simulink model "ovap_sim"  (R2025a)
settings: Solver=FixedStepAuto  StartTime=0.0  StopTime=100  FixedStep=0.002  RelTol=1e-3
undefined symbols (not defined in the file): X, Y, Z
libraries: sm_lib x88, nesl_utility x45, simulink_extras x31, slpidlib x8
(part 3 of 5)

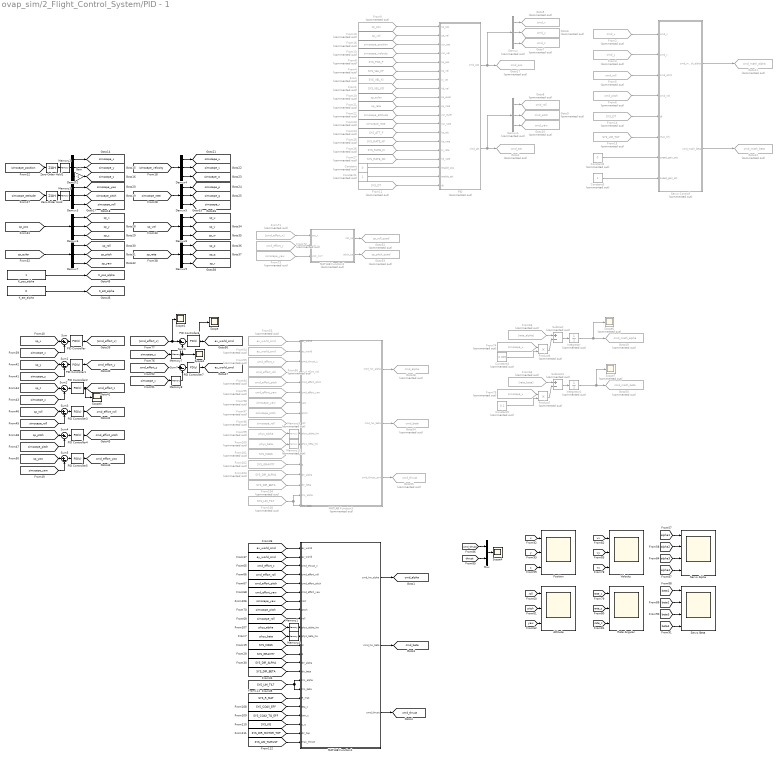
== system ovap_sim/2_Flight_Control_System/PID - 1 ==
  Attitude : Scope  NumInputPorts=3
      settings: ActiveDisplayYMinimum=-1.3426964874855616  ActiveDisplayYMaximum=11.260296121880314  DataLoggingVariableName=ScopeData17
  Constant : Constant  Commented=on  Value=0
  Constant1 : Constant  Commented=on
  Constant2 : Constant  Commented=on  Value=0
  Constant3 : Constant  Commented=on
  Constant4 : Constant  Commented=on  Value=0.005
  Constant5 : Constant  Commented=on  Value=0.1
  Demux : Demux  Commented=on  Outputs=3
  Demux1 : Demux  Commented=on  Outputs=3
  Demux{2..9} (8 alike) : Demux  Outputs=3
  From : From  Commented=on  GotoTag=SYS_VEL_KI  TagVisibility=global
  From1 : From  Commented=on  GotoTag=SYS_VEL_KD  TagVisibility=global
  From10 : From  Commented=on  GotoTag=sp_vel  TagVisibility=global
  From100 : From  Commented=on  GotoTag=phys_beta  TagVisibility=global
  From101 : From  Commented=on  GotoTag=SYS_MASS  TagVisibility=global
  From102 : From  Commented=on  GotoTag=SYS_GRAVITY  TagVisibility=global
  From103 : From  Commented=on  GotoTag=SYS_DIR_ALPHA  TagVisibility=global
  From104 : From  Commented=on  GotoTag=SYS_DIR_BETA  TagVisibility=global
  From105 : From  Commented=on  GotoTag=SYS_LIM_TILT  TagVisibility=global
  From11 : From  Commented=on  GotoTag=SYS_DT  TagVisibility=global
  From13 : From  Commented=on  GotoTag=simscape_velocity  TagVisibility=global
  From14 : From  Commented=on  GotoTag=SYS_DT  TagVisibility=global
  From15 : From  Commented=on  GotoTag=SYS_LIM_TILT  TagVisibility=global
  From16 : From  Commented=on  GotoTag=simscape_position  TagVisibility=global
  From2 : From  Commented=on  GotoTag=cmd_x  TagVisibility=global
  From20 : From  Commented=on  GotoTag=sp_euler  TagVisibility=global
  From21 : From  Commented=on  GotoTag=sp_rate  TagVisibility=global
  From22 : From  Commented=on  GotoTag=simscape_attitude  TagVisibility=global
  From23 : From  Commented=on  GotoTag=simscape_rate  TagVisibility=global
  From24 : From  Commented=on  GotoTag=SYS_ATT_P  TagVisibility=global
  From25 : From  Commented=on  GotoTag=SYS_RATE_KP  TagVisibility=global
  From26 : From  Commented=on  GotoTag=SYS_RATE_KI  TagVisibility=global
  From27 : From  Commented=on  GotoTag=SYS_RATE_KD  TagVisibility=global
  From3 : From  Commented=on  GotoTag=cmd_y  TagVisibility=global
  From4 : From  Commented=on  GotoTag=SYS_VEL_KP  TagVisibility=global
  From5 : From  Commented=on  GotoTag=cmd_roll  TagVisibility=global
  From53 : From  Commented=on  GotoTag=ax_world_cmd  TagVisibility=global
  From54 : From  Commented=on  GotoTag=ay_world_cmd  TagVisibility=global
  From55 : From  Commented=on  GotoTag=cmd_effort_z  TagVisibility=global
  From56 : From  Commented=on  GotoTag=cmd_effort_roll  TagVisibility=global
  From6 : From  Commented=on  GotoTag=cmd_pitch  TagVisibility=global
  From63 : From  Commented=on  GotoTag=rate_alpha
  From64 : From  Commented=on  GotoTag=rate_beta
  From71 : From  Commented=on  GotoTag=cmd_effort_x
  From72 : From  Commented=on  GotoTag=cmd_effort_y  TagVisibility=global
  From73 : From  Commented=on  GotoTag=simscape_yaw  TagVisibility=global
  From74 : From  Commented=on  GotoTag=simscape_u  TagVisibility=global
  From75 : From  Commented=on  GotoTag=simscape_v  TagVisibility=global
  From8 : From  Commented=on  GotoTag=SYS_POS_P  TagVisibility=global
  From9 : From  Commented=on  GotoTag=sp_pos  TagVisibility=global
  From94 : From  Commented=on  GotoTag=cmd_effort_pitch  TagVisibility=global
  From95 : From  Commented=on  GotoTag=cmd_effort_yaw  TagVisibility=global
  From96 : From  Commented=on  GotoTag=simscape_roll  TagVisibility=global
  From97 : From  Commented=on  GotoTag=simscape_pitch  TagVisibility=global
  From98 : From  Commented=on  GotoTag=simscape_yaw  TagVisibility=global
  From99 : From  Commented=on  GotoTag=phys_alpha  TagVisibility=global
  Gain : Gain  Gain=-1
  Goto10 : Goto  Commented=on  GotoTag=cmd_yaw  TagVisibility=global
  Goto11 : Goto  Commented=on  GotoTag=cmd_math_alpha  TagVisibility=global
  Goto12 : Goto  Commented=on  GotoTag=cmd_math_beta  TagVisibility=global
  Goto17 : Goto  Commented=on  GotoTag=cmd_pos  TagVisibility=global
  Goto2 : Goto  Commented=on  GotoTag=cmd_att  TagVisibility=global
  Goto48 : Goto  Commented=on  GotoTag=cmd_alpha  TagVisibility=global
  Goto49 : Goto  Commented=on  GotoTag=cmd_math_alpha  TagVisibility=global
  Goto5 : Goto  Commented=on  GotoTag=cmd_x  TagVisibility=global
  Goto50 : Goto  Commented=on  GotoTag=cmd_math_beta  TagVisibility=global
  Goto52 : Goto  Commented=on  GotoTag=sp_roll_quad  TagVisibility=global
  Goto53 : Goto  Commented=on  GotoTag=sp_pitch_quad  TagVisibility=global
  Goto54 : Goto  Commented=on  GotoTag=cmd_beta  TagVisibility=global
  Goto55 : Goto  Commented=on  GotoTag=cmd_thrust  TagVisibility=global
  Goto6 : Goto  Commented=on  GotoTag=cmd_y  TagVisibility=global
  Goto7 : Goto  Commented=on  GotoTag=cmd_z  TagVisibility=global
  Goto8 : Goto  Commented=on  GotoTag=cmd_roll  TagVisibility=global
  Goto9 : Goto  Commented=on  GotoTag=cmd_pitch  TagVisibility=global
  Integrator : Integrator  Commented=on  LimitOutput=on  UpperSaturationLimit=5*pi/180  LowerSaturationLimit=-5*pi/180
  Integrator1 : Integrator  Commented=on  LimitOutput=on  UpperSaturationLimit=5  LowerSaturationLimit=-5
  K_att_alpha : Constant  Value=0
  K_pos_alpha : Constant
  MATLAB Function1 : MATLAB Function  TreatAsAtomicUnit=on
  MATLAB Function2 : MATLAB Function  Commented=on  TreatAsAtomicUnit=on
  MATLAB Function3 : MATLAB Function  Commented=on  TreatAsAtomicUnit=on
  Memory{1..4,7..8} (6 alike) : Memory
  Memory10 : Memory  Commented=on
  Memory9 : Memory  Commented=on
  Mux : Mux  Inputs=2
  PID : MATLAB Function  Commented=on  TreatAsAtomicUnit=on
  PID Controller : slpidlib/PID Controller  Controller=PID  Form=Parallel  TimeDomain=Discrete-time  UseExternalTs=off  SampleTime=0.002  IntegratorMethod=Forward Euler  FilterMethod=Forward Euler  ControllerParametersSource=internal  P=15  I=0.0001  UseKiTs=off  D=27  UseExternalDerivativeSource=off  N=100  UseFilter=on  TunerSelectOption=Transfer Function Based (PID Tuner App)  InitialConditionSource=internal  InitialConditionForIntegrator=0  InitialConditionForFilter=0  DifferentiatorICPrevScaledInput=0  ExternalReset=none  TrackingMode=off  Kt=1  LimitOutput=off  SatLimitsSource=internal  UpperSaturationLimit=1  LowerSaturationLimit=-1  LinearizeAsGain=off  AntiWindupMode=clamping  Kb=1  LimitIntegrator=off  UpperIntegratorSaturationLimit=inf  LowerIntegratorSaturationLimit=-inf  POutMin=[]  POutMax=[]  IOutMin=[]  IOutMax=[]  DOutMin=[]  DOutMax=[]  NOutMin=[]  NOutMax=[]  SumOutMin=[]  SumOutMax=[]  SaturationOutMin=[]  SaturationOutMax=[]  PParamMin=[]  PParamMax=[]  IParamMin=[]  IParamMax=[]  DParamMin=[]  DParamMax=[]  NParamMin=[]  NParamMax=[]  KbParamMin=[]  KbParamMax=[]  KtParamMin=[]  KtParamMax=[]  KbOutMin=[]  KbOutMax=[]  KtOutMin=[]  KtOutMax=[]  IntegratorOutMin=[]  IntegratorOutMax=[]  FilterOutMin=[]  FilterOutMax=[]  SumI1OutMin=[]  SumI1OutMax=[]  SumI2OutMin=[]  SumI2OutMax=[]  SumI3OutMin=[]  SumI3OutMax=[]  SumI4OutMin=[]  SumI4OutMax=[]  SumDOutMin=[]  SumDOutMax=[]  DifferentiatorOutMin=[]  DifferentiatorOutMax=[]  FilterDiffOutCoefMin=[]  FilterDiffOutCoefMax=[]  ReciprocalOutMin=[]  ReciprocalOutMax=[]  SumDenOutMin=[]  SumDenOutMax=[]  SumNumOutMin=[]  SumNumOutMax=[]  DivideOutMin=[]  DivideOutMax=[]  UdiffTsProdOutMin=[]  UdiffTsProdOutMax=[]  NTsProdOutMin=[]  NTsProdOutMax=[]  UintegralTsProdOutMin=[]  UintegralTsProdOutMax=[]  UngainTsProdOutMin=[]  UngainTsProdOutMax=[]  ClampingZeroOutDataTypeStr=Inherit: Inherit via back propagation  ClampingZeroOutMin=[]  ClampingZeroOutMax=[]  FilterDenConstantOutDataTypeStr=Inherit: Inherit via back propagation  FilterDenConstantOutMin=[]  FilterDenConstantOutMax=[]  PCopyOutDataTypeStr=Inherit: Inherit via back propagation  PCopyOutMin=[]  PCopyOutMax=[]  NCopyOutDataTypeStr=Inherit: Inherit via back propagation  NCopyOutMin=[]  NCopyOutMax=[]  IntegratorContinuousStateAttributes=''  IntegratorStateMustResolveToSignalObject=off  IntegratorRTWStateStorageClass=Auto  FilterContinuousStateAttributes=''  FilterStateMustResolveToSignalObject=off  FilterRTWStateStorageClass=Auto  ParallelPVariant=InternalParameters  IdealPVariant=Disabled  IVariant=InternalParameters  DVariant=InternalParameters  IntegratorVariant=Discrete  SatVariant=Disabled  AWVariant=Passthrough  PCopyVariant=Disabled  TRVariant=Disabled  FdbkBlocksVariant=Forward  IdealPFdbkVariant=Disabled  SatFdbkVariant=Disabled  DerivativeFilterVariant=ForwardEulerFilter  NVariant=InternalParameters  NCopyVariant=Disabled  FilterICVariant=InternalICsFilter  IntegratorICVariant=InternalICs  ExternalResetVariant=Disabled  TRSumVariant=Passthrough  SumFdbkVariant=Disabled  SumVariant=Sum_PID  TsampFilterVariant=InternalTs  TsampNgainVariant=Passthrough  TsampIntegralVariant=Disabled_SignalSpec  ExternalSaturationOutDataTypeStr=Inherit: Same as second input  DerivativeSourceVariant=ErrorSignal  PreIntVariant=InternalPreInt
  PID Controller1 : slpidlib/PID Controller  Controller=PID  Form=Parallel  TimeDomain=Discrete-time  UseExternalTs=off  SampleTime=0.002  IntegratorMethod=Forward Euler  FilterMethod=Forward Euler  ControllerParametersSource=internal  P=3  I=0.0001  UseKiTs=off  D=0  UseExternalDerivativeSource=off  N=100  UseFilter=on  TunerSelectOption=Transfer Function Based (PID Tuner App)  InitialConditionSource=internal  InitialConditionForIntegrator=0  InitialConditionForFilter=0  DifferentiatorICPrevScaledInput=0  ExternalReset=none  TrackingMode=off  Kt=1  LimitOutput=on  SatLimitsSource=internal  UpperSaturationLimit=5  LowerSaturationLimit=-5  LinearizeAsGain=on  AntiWindupMode=clamping  Kb=1  LimitIntegrator=off  UpperIntegratorSaturationLimit=inf  LowerIntegratorSaturationLimit=-inf  POutMin=[]  POutMax=[]  IOutMin=[]  IOutMax=[]  DOutMin=[]  DOutMax=[]  NOutMin=[]  NOutMax=[]  SumOutMin=[]  SumOutMax=[]  SaturationOutMin=[]  SaturationOutMax=[]  PParamMin=[]  PParamMax=[]  IParamMin=[]  IParamMax=[]  DParamMin=[]  DParamMax=[]  NParamMin=[]  NParamMax=[]  KbParamMin=[]  KbParamMax=[]  KtParamMin=[]  KtParamMax=[]  KbOutMin=[]  KbOutMax=[]  KtOutMin=[]  KtOutMax=[]  IntegratorOutMin=[]  IntegratorOutMax=[]  FilterOutMin=[]  FilterOutMax=[]  SumI1OutMin=[]  SumI1OutMax=[]  SumI2OutMin=[]  SumI2OutMax=[]  SumI3OutMin=[]  SumI3OutMax=[]  SumI4OutMin=[]  SumI4OutMax=[]  SumDOutMin=[]  SumDOutMax=[]  DifferentiatorOutMin=[]  DifferentiatorOutMax=[]  FilterDiffOutCoefMin=[]  FilterDiffOutCoefMax=[]  ReciprocalOutMin=[]  ReciprocalOutMax=[]  SumDenOutMin=[]  SumDenOutMax=[]  SumNumOutMin=[]  SumNumOutMax=[]  DivideOutMin=[]  DivideOutMax=[]  UdiffTsProdOutMin=[]  UdiffTsProdOutMax=[]  NTsProdOutMin=[]  NTsProdOutMax=[]  UintegralTsProdOutMin=[]  UintegralTsProdOutMax=[]  UngainTsProdOutMin=[]  UngainTsProdOutMax=[]  ClampingZeroOutDataTypeStr=Inherit: Inherit via back propagation  ClampingZeroOutMin=[]  ClampingZeroOutMax=[]  FilterDenConstantOutDataTypeStr=Inherit: Inherit via back propagation  FilterDenConstantOutMin=[]  FilterDenConstantOutMax=[]  PCopyOutDataTypeStr=Inherit: Inherit via back propagation  PCopyOutMin=[]  PCopyOutMax=[]  NCopyOutDataTypeStr=Inherit: Inherit via back propagation  NCopyOutMin=[]  NCopyOutMax=[]  IntegratorContinuousStateAttributes=''  IntegratorStateMustResolveToSignalObject=off  IntegratorRTWStateStorageClass=Auto  FilterContinuousStateAttributes=''  FilterStateMustResolveToSignalObject=off  FilterRTWStateStorageClass=Auto  ParallelPVariant=InternalParameters  IdealPVariant=Disabled  IVariant=InternalParameters  DVariant=InternalParameters  IntegratorVariant=Discrete  SatVariant=Enabled  AWVariant=DiscClampingParallel  PCopyVariant=Disabled  TRVariant=Disabled  FdbkBlocksVariant=Forward  IdealPFdbkVariant=Disabled  SatFdbkVariant=Disabled  DerivativeFilterVariant=ForwardEulerFilter  NVariant=InternalParameters  NCopyVariant=Disabled  FilterICVariant=InternalICsFilter  IntegratorICVariant=InternalICs  ExternalResetVariant=Disabled  TRSumVariant=Passthrough  SumFdbkVariant=Disabled  SumVariant=Sum_PID  TsampFilterVariant=InternalTs  TsampNgainVariant=Passthrough  TsampIntegralVariant=Disabled_SignalSpec  ExternalSaturationOutDataTypeStr=Inherit: Same as second input  DerivativeSourceVariant=ErrorSignal  PreIntVariant=InternalPreInt
  PID Controller2 : slpidlib/PID Controller  Controller=PID  Form=Parallel  TimeDomain=Discrete-time  UseExternalTs=off  SampleTime=0.002  IntegratorMethod=Forward Euler  FilterMethod=Forward Euler  ControllerParametersSource=internal  P=3  I=0.0001  UseKiTs=off  D=9.5  UseExternalDerivativeSource=off  N=100  UseFilter=on  TunerSelectOption=Transfer Function Based (PID Tuner App)  InitialConditionSource=internal  InitialConditionForIntegrator=0  InitialConditionForFilter=0  DifferentiatorICPrevScaledInput=0  ExternalReset=none  TrackingMode=off  Kt=1  LimitOutput=on  SatLimitsSource=internal  UpperSaturationLimit=5  LowerSaturationLimit=-5  LinearizeAsGain=on  AntiWindupMode=clamping  Kb=1  LimitIntegrator=off  UpperIntegratorSaturationLimit=inf  LowerIntegratorSaturationLimit=-inf  POutMin=[]  POutMax=[]  IOutMin=[]  IOutMax=[]  DOutMin=[]  DOutMax=[]  NOutMin=[]  NOutMax=[]  SumOutMin=[]  SumOutMax=[]  SaturationOutMin=[]  SaturationOutMax=[]  PParamMin=[]  PParamMax=[]  IParamMin=[]  IParamMax=[]  DParamMin=[]  DParamMax=[]  NParamMin=[]  NParamMax=[]  KbParamMin=[]  KbParamMax=[]  KtParamMin=[]  KtParamMax=[]  KbOutMin=[]  KbOutMax=[]  KtOutMin=[]  KtOutMax=[]  IntegratorOutMin=[]  IntegratorOutMax=[]  FilterOutMin=[]  FilterOutMax=[]  SumI1OutMin=[]  SumI1OutMax=[]  SumI2OutMin=[]  SumI2OutMax=[]  SumI3OutMin=[]  SumI3OutMax=[]  SumI4OutMin=[]  SumI4OutMax=[]  SumDOutMin=[]  SumDOutMax=[]  DifferentiatorOutMin=[]  DifferentiatorOutMax=[]  FilterDiffOutCoefMin=[]  FilterDiffOutCoefMax=[]  ReciprocalOutMin=[]  ReciprocalOutMax=[]  SumDenOutMin=[]  SumDenOutMax=[]  SumNumOutMin=[]  SumNumOutMax=[]  DivideOutMin=[]  DivideOutMax=[]  UdiffTsProdOutMin=[]  UdiffTsProdOutMax=[]  NTsProdOutMin=[]  NTsProdOutMax=[]  UintegralTsProdOutMin=[]  UintegralTsProdOutMax=[]  UngainTsProdOutMin=[]  UngainTsProdOutMax=[]  ClampingZeroOutDataTypeStr=Inherit: Inherit via back propagation  ClampingZeroOutMin=[]  ClampingZeroOutMax=[]  FilterDenConstantOutDataTypeStr=Inherit: Inherit via back propagation  FilterDenConstantOutMin=[]  FilterDenConstantOutMax=[]  PCopyOutDataTypeStr=Inherit: Inherit via back propagation  PCopyOutMin=[]  PCopyOutMax=[]  NCopyOutDataTypeStr=Inherit: Inherit via back propagation  NCopyOutMin=[]  NCopyOutMax=[]  IntegratorContinuousStateAttributes=''  IntegratorStateMustResolveToSignalObject=off  IntegratorRTWStateStorageClass=Auto  FilterContinuousStateAttributes=''  FilterStateMustResolveToSignalObject=off  FilterRTWStateStorageClass=Auto  ParallelPVariant=InternalParameters  IdealPVariant=Disabled  IVariant=InternalParameters  DVariant=InternalParameters  IntegratorVariant=Discrete  SatVariant=Enabled  AWVariant=DiscClampingParallel  PCopyVariant=Disabled  TRVariant=Disabled  FdbkBlocksVariant=Forward  IdealPFdbkVariant=Disabled  SatFdbkVariant=Disabled  DerivativeFilterVariant=ForwardEulerFilter  NVariant=InternalParameters  NCopyVariant=Disabled  FilterICVariant=InternalICsFilter  IntegratorICVariant=InternalICs  ExternalResetVariant=Disabled  TRSumVariant=Passthrough  SumFdbkVariant=Disabled  SumVariant=Sum_PID  TsampFilterVariant=InternalTs  TsampNgainVariant=Passthrough  TsampIntegralVariant=Disabled_SignalSpec  ExternalSaturationOutDataTypeStr=Inherit: Same as second input  DerivativeSourceVariant=ErrorSignal  PreIntVariant=InternalPreInt
  PID Controller3 : slpidlib/PID Controller  Controller=PID  Form=Parallel  TimeDomain=Discrete-time  UseExternalTs=off  SampleTime=0.002  IntegratorMethod=Forward Euler  FilterMethod=Forward Euler  ControllerParametersSource=internal  P=0.05  I=0.0001  UseKiTs=off  D=0.4  UseExternalDerivativeSource=off  N=100  UseFilter=on  TunerSelectOption=Transfer Function Based (PID Tuner App)  InitialConditionSource=internal  InitialConditionForIntegrator=0  InitialConditionForFilter=0  DifferentiatorICPrevScaledInput=0  ExternalReset=none  TrackingMode=off  Kt=1  LimitOutput=on  SatLimitsSource=internal  UpperSaturationLimit=5  LowerSaturationLimit=-5  LinearizeAsGain=on  AntiWindupMode=none  Kb=1  LimitIntegrator=off  UpperIntegratorSaturationLimit=inf  LowerIntegratorSaturationLimit=-inf  POutMin=[]  POutMax=[]  IOutMin=[]  IOutMax=[]  DOutMin=[]  DOutMax=[]  NOutMin=[]  NOutMax=[]  SumOutMin=[]  SumOutMax=[]  SaturationOutMin=[]  SaturationOutMax=[]  PParamMin=[]  PParamMax=[]  IParamMin=[]  IParamMax=[]  DParamMin=[]  DParamMax=[]  NParamMin=[]  NParamMax=[]  KbParamMin=[]  KbParamMax=[]  KtParamMin=[]  KtParamMax=[]  KbOutMin=[]  KbOutMax=[]  KtOutMin=[]  KtOutMax=[]  IntegratorOutMin=[]  IntegratorOutMax=[]  FilterOutMin=[]  FilterOutMax=[]  SumI1OutMin=[]  SumI1OutMax=[]  SumI2OutMin=[]  SumI2OutMax=[]  SumI3OutMin=[]  SumI3OutMax=[]  SumI4OutMin=[]  SumI4OutMax=[]  SumDOutMin=[]  SumDOutMax=[]  DifferentiatorOutMin=[]  DifferentiatorOutMax=[]  FilterDiffOutCoefMin=[]  FilterDiffOutCoefMax=[]  ReciprocalOutMin=[]  ReciprocalOutMax=[]  SumDenOutMin=[]  SumDenOutMax=[]  SumNumOutMin=[]  SumNumOutMax=[]  DivideOutMin=[]  DivideOutMax=[]  UdiffTsProdOutMin=[]  UdiffTsProdOutMax=[]  NTsProdOutMin=[]  NTsProdOutMax=[]  UintegralTsProdOutMin=[]  UintegralTsProdOutMax=[]  UngainTsProdOutMin=[]  UngainTsProdOutMax=[]  ClampingZeroOutDataTypeStr=Inherit: Inherit via back propagation  ClampingZeroOutMin=[]  ClampingZeroOutMax=[]  FilterDenConstantOutDataTypeStr=Inherit: Inherit via back propagation  FilterDenConstantOutMin=[]  FilterDenConstantOutMax=[]  PCopyOutDataTypeStr=Inherit: Inherit via back propagation  PCopyOutMin=[]  PCopyOutMax=[]  NCopyOutDataTypeStr=Inherit: Inherit via back propagation  NCopyOutMin=[]  NCopyOutMax=[]  IntegratorContinuousStateAttributes=''  IntegratorStateMustResolveToSignalObject=off  IntegratorRTWStateStorageClass=Auto  FilterContinuousStateAttributes=''  FilterStateMustResolveToSignalObject=off  FilterRTWStateStorageClass=Auto  ParallelPVariant=InternalParameters  IdealPVariant=Disabled  IVariant=InternalParameters  DVariant=InternalParameters  IntegratorVariant=Discrete  SatVariant=Enabled  AWVariant=Passthrough  PCopyVariant=Disabled  TRVariant=Disabled  FdbkBlocksVariant=Forward  IdealPFdbkVariant=Disabled  SatFdbkVariant=Disabled  DerivativeFilterVariant=ForwardEulerFilter  NVariant=InternalParameters  NCopyVariant=Disabled  FilterICVariant=InternalICsFilter  IntegratorICVariant=InternalICs  ExternalResetVariant=Disabled  TRSumVariant=Passthrough  SumFdbkVariant=Disabled  SumVariant=Sum_PID  TsampFilterVariant=InternalTs  TsampNgainVariant=Passthrough  TsampIntegralVariant=Disabled_SignalSpec  ExternalSaturationOutDataTypeStr=Inherit: Same as second input  DerivativeSourceVariant=ErrorSignal  PreIntVariant=InternalPreInt
  PID Controller4 : slpidlib/PID Controller  Controller=PID  Form=Parallel  TimeDomain=Discrete-time  UseExternalTs=off  SampleTime=0.002  IntegratorMethod=Forward Euler  FilterMethod=Forward Euler  ControllerParametersSource=internal  P=0.06  I=0.00012  UseKiTs=off  D=0.68  UseExternalDerivativeSource=off  N=100  UseFilter=on  TunerSelectOption=Transfer Function Based (PID Tuner App)  InitialConditionSource=internal  InitialConditionForIntegrator=0  InitialConditionForFilter=0  DifferentiatorICPrevScaledInput=0  ExternalReset=none  TrackingMode=off  Kt=1  LimitOutput=on  SatLimitsSource=internal  UpperSaturationLimit=5  LowerSaturationLimit=-5  LinearizeAsGain=on  AntiWindupMode=none  Kb=1  LimitIntegrator=off  UpperIntegratorSaturationLimit=inf  LowerIntegratorSaturationLimit=-inf  POutMin=[]  POutMax=[]  IOutMin=[]  IOutMax=[]  DOutMin=[]  DOutMax=[]  NOutMin=[]  NOutMax=[]  SumOutMin=[]  SumOutMax=[]  SaturationOutMin=[]  SaturationOutMax=[]  PParamMin=[]  PParamMax=[]  IParamMin=[]  IParamMax=[]  DParamMin=[]  DParamMax=[]  NParamMin=[]  NParamMax=[]  KbParamMin=[]  KbParamMax=[]  KtParamMin=[]  KtParamMax=[]  KbOutMin=[]  KbOutMax=[]  KtOutMin=[]  KtOutMax=[]  IntegratorOutMin=[]  IntegratorOutMax=[]  FilterOutMin=[]  FilterOutMax=[]  SumI1OutMin=[]  SumI1OutMax=[]  SumI2OutMin=[]  SumI2OutMax=[]  SumI3OutMin=[]  SumI3OutMax=[]  SumI4OutMin=[]  SumI4OutMax=[]  SumDOutMin=[]  SumDOutMax=[]  DifferentiatorOutMin=[]  DifferentiatorOutMax=[]  FilterDiffOutCoefMin=[]  FilterDiffOutCoefMax=[]  ReciprocalOutMin=[]  ReciprocalOutMax=[]  SumDenOutMin=[]  SumDenOutMax=[]  SumNumOutMin=[]  SumNumOutMax=[]  DivideOutMin=[]  DivideOutMax=[]  UdiffTsProdOutMin=[]  UdiffTsProdOutMax=[]  NTsProdOutMin=[]  NTsProdOutMax=[]  UintegralTsProdOutMin=[]  UintegralTsProdOutMax=[]  UngainTsProdOutMin=[]  UngainTsProdOutMax=[]  ClampingZeroOutDataTypeStr=Inherit: Inherit via back propagation  ClampingZeroOutMin=[]  ClampingZeroOutMax=[]  FilterDenConstantOutDataTypeStr=Inherit: Inherit via back propagation  FilterDenConstantOutMin=[]  FilterDenConstantOutMax=[]  PCopyOutDataTypeStr=Inherit: Inherit via back propagation  PCopyOutMin=[]  PCopyOutMax=[]  NCopyOutDataTypeStr=Inherit: Inherit via back propagation  NCopyOutMin=[]  NCopyOutMax=[]  IntegratorContinuousStateAttributes=''  IntegratorStateMustResolveToSignalObject=off  IntegratorRTWStateStorageClass=Auto  FilterContinuousStateAttributes=''  FilterStateMustResolveToSignalObject=off  FilterRTWStateStorageClass=Auto  ParallelPVariant=InternalParameters  IdealPVariant=Disabled  IVariant=InternalParameters  DVariant=InternalParameters  IntegratorVariant=Discrete  SatVariant=Enabled  AWVariant=Passthrough  PCopyVariant=Disabled  TRVariant=Disabled  FdbkBlocksVariant=Forward  IdealPFdbkVariant=Disabled  SatFdbkVariant=Disabled  DerivativeFilterVariant=ForwardEulerFilter  NVariant=InternalParameters  NCopyVariant=Disabled  FilterICVariant=InternalICsFilter  IntegratorICVariant=InternalICs  ExternalResetVariant=Disabled  TRSumVariant=Passthrough  SumFdbkVariant=Disabled  SumVariant=Sum_PID  TsampFilterVariant=InternalTs  TsampNgainVariant=Passthrough  TsampIntegralVariant=Disabled_SignalSpec  ExternalSaturationOutDataTypeStr=Inherit: Same as second input  DerivativeSourceVariant=ErrorSignal  PreIntVariant=InternalPreInt
  PID Controller5 : slpidlib/PID Controller  Controller=PID  Form=Parallel  TimeDomain=Discrete-time  UseExternalTs=off  SampleTime=0.002  IntegratorMethod=Forward Euler  FilterMethod=Forward Euler  ControllerParametersSource=internal  P=2  I=0.0001  UseKiTs=off  D=16  UseExternalDerivativeSource=off  N=100  UseFilter=on  TunerSelectOption=Transfer Function Based (PID Tuner App)  InitialConditionSource=internal  InitialConditionForIntegrator=0  InitialConditionForFilter=0  DifferentiatorICPrevScaledInput=0  ExternalReset=none  TrackingMode=off  Kt=1  LimitOutput=on  SatLimitsSource=internal  UpperSaturationLimit=5  LowerSaturationLimit=-5  LinearizeAsGain=on  AntiWindupMode=none  Kb=1  LimitIntegrator=off  UpperIntegratorSaturationLimit=inf  LowerIntegratorSaturationLimit=-inf  POutMin=[]  POutMax=[]  IOutMin=[]  IOutMax=[]  DOutMin=[]  DOutMax=[]  NOutMin=[]  NOutMax=[]  SumOutMin=[]  SumOutMax=[]  SaturationOutMin=[]  SaturationOutMax=[]  PParamMin=[]  PParamMax=[]  IParamMin=[]  IParamMax=[]  DParamMin=[]  DParamMax=[]  NParamMin=[]  NParamMax=[]  KbParamMin=[]  KbParamMax=[]  KtParamMin=[]  KtParamMax=[]  KbOutMin=[]  KbOutMax=[]  KtOutMin=[]  KtOutMax=[]  IntegratorOutMin=[]  IntegratorOutMax=[]  FilterOutMin=[]  FilterOutMax=[]  SumI1OutMin=[]  SumI1OutMax=[]  SumI2OutMin=[]  SumI2OutMax=[]  SumI3OutMin=[]  SumI3OutMax=[]  SumI4OutMin=[]  SumI4OutMax=[]  SumDOutMin=[]  SumDOutMax=[]  DifferentiatorOutMin=[]  DifferentiatorOutMax=[]  FilterDiffOutCoefMin=[]  FilterDiffOutCoefMax=[]  ReciprocalOutMin=[]  ReciprocalOutMax=[]  SumDenOutMin=[]  SumDenOutMax=[]  SumNumOutMin=[]  SumNumOutMax=[]  DivideOutMin=[]  DivideOutMax=[]  UdiffTsProdOutMin=[]  UdiffTsProdOutMax=[]  NTsProdOutMin=[]  NTsProdOutMax=[]  UintegralTsProdOutMin=[]  UintegralTsProdOutMax=[]  UngainTsProdOutMin=[]  UngainTsProdOutMax=[]  ClampingZeroOutDataTypeStr=Inherit: Inherit via back propagation  ClampingZeroOutMin=[]  ClampingZeroOutMax=[]  FilterDenConstantOutDataTypeStr=Inherit: Inherit via back propagation  FilterDenConstantOutMin=[]  FilterDenConstantOutMax=[]  PCopyOutDataTypeStr=Inherit: Inherit via back propagation  PCopyOutMin=[]  PCopyOutMax=[]  NCopyOutDataTypeStr=Inherit: Inherit via back propagation  NCopyOutMin=[]  NCopyOutMax=[]  IntegratorContinuousStateAttributes=''  IntegratorStateMustResolveToSignalObject=off  IntegratorRTWStateStorageClass=Auto  FilterContinuousStateAttributes=''  FilterStateMustResolveToSignalObject=off  FilterRTWStateStorageClass=Auto  ParallelPVariant=InternalParameters  IdealPVariant=Disabled  IVariant=InternalParameters  DVariant=InternalParameters  IntegratorVariant=Discrete  SatVariant=Enabled  AWVariant=Passthrough  PCopyVariant=Disabled  TRVariant=Disabled  FdbkBlocksVariant=Forward  IdealPFdbkVariant=Disabled  SatFdbkVariant=Disabled  DerivativeFilterVariant=ForwardEulerFilter  NVariant=InternalParameters  NCopyVariant=Disabled  FilterICVariant=InternalICsFilter  IntegratorICVariant=InternalICs  ExternalResetVariant=Disabled  TRSumVariant=Passthrough  SumFdbkVariant=Disabled  SumVariant=Sum_PID  TsampFilterVariant=InternalTs  TsampNgainVariant=Passthrough  TsampIntegralVariant=Disabled_SignalSpec  ExternalSaturationOutDataTypeStr=Inherit: Same as second input  DerivativeSourceVariant=ErrorSignal  PreIntVariant=InternalPreInt
  PID Controller6 : slpidlib/PID Controller  Controller=PD  Form=Parallel  TimeDomain=Discrete-time  UseExternalTs=off  SampleTime=0.002  IntegratorMethod=Forward Euler  FilterMethod=Forward Euler  ControllerParametersSource=internal  P=1  I=0  UseKiTs=off  D=0.05  UseExternalDerivativeSource=off  N=100  UseFilter=on  TunerSelectOption=Transfer Function Based (PID Tuner App)  InitialConditionSource=internal  InitialConditionForIntegrator=0  InitialConditionForFilter=0  DifferentiatorICPrevScaledInput=0  ExternalReset=none  TrackingMode=off  Kt=1  LimitOutput=on  SatLimitsSource=internal  UpperSaturationLimit=3  LowerSaturationLimit=-3  LinearizeAsGain=off  AntiWindupMode=clamping  Kb=1  LimitIntegrator=off  UpperIntegratorSaturationLimit=inf  LowerIntegratorSaturationLimit=-inf  POutMin=[]  POutMax=[]  IOutMin=[]  IOutMax=[]  DOutMin=[]  DOutMax=[]  NOutMin=[]  NOutMax=[]  SumOutMin=[]  SumOutMax=[]  SaturationOutMin=[]  SaturationOutMax=[]  PParamMin=[]  PParamMax=[]  IParamMin=[]  IParamMax=[]  DParamMin=[]  DParamMax=[]  NParamMin=[]  NParamMax=[]  KbParamMin=[]  KbParamMax=[]  KtParamMin=[]  KtParamMax=[]  KbOutMin=[]  KbOutMax=[]  KtOutMin=[]  KtOutMax=[]  IntegratorOutMin=[]  IntegratorOutMax=[]  FilterOutMin=[]  FilterOutMax=[]  SumI1OutMin=[]  SumI1OutMax=[]  SumI2OutMin=[]  SumI2OutMax=[]  SumI3OutMin=[]  SumI3OutMax=[]  SumI4OutMin=[]  SumI4OutMax=[]  SumDOutMin=[]  SumDOutMax=[]  DifferentiatorOutMin=[]  DifferentiatorOutMax=[]  FilterDiffOutCoefMin=[]  FilterDiffOutCoefMax=[]  ReciprocalOutMin=[]  ReciprocalOutMax=[]  SumDenOutMin=[]  SumDenOutMax=[]  SumNumOutMin=[]  SumNumOutMax=[]  DivideOutMin=[]  DivideOutMax=[]  UdiffTsProdOutMin=[]  UdiffTsProdOutMax=[]  NTsProdOutMin=[]  NTsProdOutMax=[]  UintegralTsProdOutMin=[]  UintegralTsProdOutMax=[]  UngainTsProdOutMin=[]  UngainTsProdOutMax=[]  ClampingZeroOutDataTypeStr=Inherit: Inherit via back propagation  ClampingZeroOutMin=[]  ClampingZeroOutMax=[]  FilterDenConstantOutDataTypeStr=Inherit: Inherit via back propagation  FilterDenConstantOutMin=[]  FilterDenConstantOutMax=[]  PCopyOutDataTypeStr=Inherit: Inherit via back propagation  PCopyOutMin=[]  PCopyOutMax=[]  NCopyOutDataTypeStr=Inherit: Inherit via back propagation  NCopyOutMin=[]  NCopyOutMax=[]  IntegratorContinuousStateAttributes=''  IntegratorStateMustResolveToSignalObject=off  IntegratorRTWStateStorageClass=Auto  FilterContinuousStateAttributes=''  FilterStateMustResolveToSignalObject=off  FilterRTWStateStorageClass=Auto  ParallelPVariant=InternalParameters  IdealPVariant=Disabled  IVariant=Disabled  DVariant=InternalParameters  IntegratorVariant=Disabled  SatVariant=Enabled  AWVariant=Disabled  PCopyVariant=Disabled  TRVariant=Disabled  FdbkBlocksVariant=Forward  IdealPFdbkVariant=Disabled  SatFdbkVariant=Disabled  DerivativeFilterVariant=ForwardEulerFilter  NVariant=InternalParameters  NCopyVariant=Disabled  FilterICVariant=InternalICsFilter  IntegratorICVariant=Disabled  ExternalResetVariant=Disabled  TRSumVariant=Passthrough  SumFdbkVariant=Disabled  SumVariant=Sum_PD  TsampFilterVariant=InternalTs  TsampNgainVariant=Passthrough  TsampIntegralVariant=Disabled_SignalSpec  ExternalSaturationOutDataTypeStr=Inherit: Same as second input  DerivativeSourceVariant=ErrorSignal  PreIntVariant=InternalPreInt
  PID Controller7 : slpidlib/PID Controller  Controller=PD  Form=Parallel  TimeDomain=Discrete-time  UseExternalTs=off  SampleTime=0.002  IntegratorMethod=Forward Euler  FilterMethod=Forward Euler  ControllerParametersSource=internal  P=1  I=0  UseKiTs=off  D=0  UseExternalDerivativeSource=off  N=100  UseFilter=on  TunerSelectOption=Transfer Function Based (PID Tuner App)  InitialConditionSource=internal  InitialConditionForIntegrator=0  InitialConditionForFilter=0  DifferentiatorICPrevScaledInput=0  ExternalReset=none  TrackingMode=off  Kt=1  LimitOutput=on  SatLimitsSource=internal  UpperSaturationLimit=3  LowerSaturationLimit=-3  LinearizeAsGain=off  AntiWindupMode=clamping  Kb=1  LimitIntegrator=off  UpperIntegratorSaturationLimit=inf  LowerIntegratorSaturationLimit=-inf  POutMin=[]  POutMax=[]  IOutMin=[]  IOutMax=[]  DOutMin=[]  DOutMax=[]  NOutMin=[]  NOutMax=[]  SumOutMin=[]  SumOutMax=[]  SaturationOutMin=[]  SaturationOutMax=[]  PParamMin=[]  PParamMax=[]  IParamMin=[]  IParamMax=[]  DParamMin=[]  DParamMax=[]  NParamMin=[]  NParamMax=[]  KbParamMin=[]  KbParamMax=[]  KtParamMin=[]  KtParamMax=[]  KbOutMin=[]  KbOutMax=[]  KtOutMin=[]  KtOutMax=[]  IntegratorOutMin=[]  IntegratorOutMax=[]  FilterOutMin=[]  FilterOutMax=[]  SumI1OutMin=[]  SumI1OutMax=[]  SumI2OutMin=[]  SumI2OutMax=[]  SumI3OutMin=[]  SumI3OutMax=[]  SumI4OutMin=[]  SumI4OutMax=[]  SumDOutMin=[]  SumDOutMax=[]  DifferentiatorOutMin=[]  DifferentiatorOutMax=[]  FilterDiffOutCoefMin=[]  FilterDiffOutCoefMax=[]  ReciprocalOutMin=[]  ReciprocalOutMax=[]  SumDenOutMin=[]  SumDenOutMax=[]  SumNumOutMin=[]  SumNumOutMax=[]  DivideOutMin=[]  DivideOutMax=[]  UdiffTsProdOutMin=[]  UdiffTsProdOutMax=[]  NTsProdOutMin=[]  NTsProdOutMax=[]  UintegralTsProdOutMin=[]  UintegralTsProdOutMax=[]  UngainTsProdOutMin=[]  UngainTsProdOutMax=[]  ClampingZeroOutDataTypeStr=Inherit: Inherit via back propagation  ClampingZeroOutMin=[]  ClampingZeroOutMax=[]  FilterDenConstantOutDataTypeStr=Inherit: Inherit via back propagation  FilterDenConstantOutMin=[]  FilterDenConstantOutMax=[]  PCopyOutDataTypeStr=Inherit: Inherit via back propagation  PCopyOutMin=[]  PCopyOutMax=[]  NCopyOutDataTypeStr=Inherit: Inherit via back propagation  NCopyOutMin=[]  NCopyOutMax=[]  IntegratorContinuousStateAttributes=''  IntegratorStateMustResolveToSignalObject=off  IntegratorRTWStateStorageClass=Auto  FilterContinuousStateAttributes=''  FilterStateMustResolveToSignalObject=off  FilterRTWStateStorageClass=Auto  ParallelPVariant=InternalParameters  IdealPVariant=Disabled  IVariant=Disabled  DVariant=InternalParameters  IntegratorVariant=Disabled  SatVariant=Enabled  AWVariant=Disabled  PCopyVariant=Disabled  TRVariant=Disabled  FdbkBlocksVariant=Forward  IdealPFdbkVariant=Disabled  SatFdbkVariant=Disabled  DerivativeFilterVariant=ForwardEulerFilter  NVariant=InternalParameters  NCopyVariant=Disabled  FilterICVariant=InternalICsFilter  IntegratorICVariant=Disabled  ExternalResetVariant=Disabled  TRSumVariant=Passthrough  SumFdbkVariant=Disabled  SumVariant=Sum_PD  TsampFilterVariant=InternalTs  TsampNgainVariant=Passthrough  TsampIntegralVariant=Disabled_SignalSpec  ExternalSaturationOutDataTypeStr=Inherit: Same as second input  DerivativeSourceVariant=ErrorSignal  PreIntVariant=InternalPreInt
  Position : Scope  NumInputPorts=3
      settings: ActiveDisplayYMinimum=-6.792042036312667  ActiveDisplayYMaximum=11.866611237359098  DataLoggingVariableName=ScopeData18
  Product6 : Product  Commented=on
  Product7 : Product  Commented=on
  Rate Angular : Scope  NumInputPorts=3
      settings: ActiveDisplayYMinimum=-143.23944878270581  ActiveDisplayYMaximum=143.23944878270581  DataLoggingVariableName=ScopeData19
  Scope{,1..2,4..5} (5 alike) : Scope
      Scope settings: ActiveDisplayYMinimum=-3.75  ActiveDisplayYMaximum=3.75  DataLoggingVariableName=ScopeData26
      Scope1 settings: ActiveDisplayYMinimum=-1  ActiveDisplayYMaximum=1  DataLoggingVariableName=ScopeData30
      Scope2 settings: ActiveDisplayYMinimum=-7.1890173710064866  ActiveDisplayYMaximum=10.758271007819056  DataLoggingVariableName=ScopeData31
      Scope4 settings: ActiveDisplayYMinimum=-1  ActiveDisplayYMaximum=1  DataLoggingVariableName=ScopeData22
      Scope5 settings: ActiveDisplayYMinimum=-2.4275828747265744  ActiveDisplayYMaximum=5.82528698608073  DataLoggingVariableName=ScopeData33
  Scope6 : Scope  Commented=on
      settings: DataLoggingVariableName=ScopeData27
  Scope7 : Scope  Commented=on
      settings: DataLoggingVariableName=ScopeData28
  Servo Alpha : Scope  NumInputPorts=4
      settings: ActiveDisplayYMinimum=-3.9267300095298534  ActiveDisplayYMaximum=3.9256735239341554  DataLoggingVariableName=ScopeData24
  Servo Beta : Scope  NumInputPorts=4
      settings: ActiveDisplayYMinimum=-3.9267300095298534  ActiveDisplayYMaximum=3.9256735239341554  DataLoggingVariableName=ScopeData25
  Servo Controll : MATLAB Function  Commented=on  TreatAsAtomicUnit=on
  Subtract : Sum  Commented=on  Inputs=+-
  Subtract1 : Sum  Commented=on  Inputs=+-
  Sum{,1..7} (8 alike) : Sum  Inputs=|+-
  Velocity : Scope  NumInputPorts=3
      settings: ActiveDisplayYMinimum=-143.23944878270581  ActiveDisplayYMaximum=143.23944878270581  DataLoggingVariableName=ScopeData29
  Zero-Order Hold : ZeroOrderHold  SampleTime=0.002
  Zero-Order Hold1 : ZeroOrderHold  SampleTime=0.002
  tag scope: K_att_alpha=global, K_pos_alpha=global, ax_world_cmd=global, ay_world_cmd=global, cmd_alpha=global, cmd_beta=global, cmd_effort_pitch=global, cmd_effort_roll=global, cmd_effort_y=global, cmd_effort_yaw=global, cmd_effort_z=global, cmd_thrust=global, simscape_p=global, simscape_pitch=global, simscape_q=global, simscape_r=global, simscape_roll=global, simscape_u=global, simscape_v=global, simscape_w=global, simscape_x=global, simscape_y=global, simscape_yaw=global, simscape_z=global, sp_p=global, sp_pitch=global, sp_q=global, sp_r=global, sp_roll=global, sp_u=global, sp_v=global, sp_w=global, sp_x=global, sp_y=global, sp_yaw=global, sp_z=global
  wires:
  PID/1(cmd_pos) -> Demux/1, Goto17/1
  From9/1 -> PID/1(sp_pos)
  From10/1 -> PID/2(sp_vel)
  From16/1 -> PID/3(cur_pos)
  From13/1 -> PID/4(cur_vel)
  From8/1 -> PID/5(kp_pos)
  From4/1 -> PID/6(kp_vel)
  From/1 -> PID/7(ki_vel)
  From1/1 -> PID/8(kd_vel)
  From20/1 -> PID/9(sp_euler)
  From21/1 -> PID/10(sp_rate)
  From22/1 -> PID/11(cur_euler)
  From23/1 -> PID/12(cur_rate)
  From24/1 -> PID/13(kp_att)
  From25/1 -> PID/14(kp_rate)
  From26/1 -> PID/15(ki_rate)
  From27/1 -> PID/16(kd_rate)
  From11/1 -> PID/19(dt)
  Constant/1 -> PID/17(enable_pos)
  Constant1/1 -> PID/18(enable_att)
  Demux/1 -> Goto5/1
  Demux/2 -> Goto6/1
  Demux/3 -> Goto7/1
  From2/1 -> Servo Controll/1(cmd_x)
  From3/1 -> Servo Controll/2(cmd_y)
  PID/2(cmd_att) -> Demux1/1, Goto2/1
  Demux1/1 -> Goto8/1
  Demux1/2 -> Goto9/1
  Demux1/3 -> Goto10/1
  From5/1 -> Servo Controll/3(cmd_pitch)
  From6/1 -> Servo Controll/4(cmd_roll)
  From14/1 -> Servo Controll/5(dt)
  From15/1 -> Servo Controll/6(max_tilt)
  Constant2/1 -> Servo Controll/7(speed_gain_pos)
  Constant3/1 -> Servo Controll/8(speed_gain_att)
  Servo Controll/1(cmd_math_alpha) -> Goto11/1
  Servo Controll/2(cmd_math_beta) -> Goto12/1
  [simscape_position] -> Zero-Order Hold1/1
  Demux2/1 -> [simscape_x]
  Demux2/2 -> [simscape_y]
  [simscape_attitude] -> Zero-Order Hold/1
  [simscape_rate] -> Demux5/1
  Demux5/2 -> [simscape_q]
  Demux5/1 -> [simscape_p]
  Demux5/3 -> [simscape_r]
  Demux4/1 -> [simscape_u]
  [simscape_velocity] -> Demux4/1
  Demux4/2 -> [simscape_v]
  Demux4/3 -> [simscape_w]
  Demux7/1 -> [sp_roll]
  Demux7/3 -> [sp_yaw]
  Demux6/1 -> [sp_x]
  [sp_pos] -> Demux6/1
  Demux9/3 -> [sp_r]
  Demux9/1 -> [sp_p]
  Demux9/2 -> [sp_q]
  Demux8/2 -> [sp_v]
  Demux8/3 -> [sp_w]
  Demux8/1 -> [sp_u]
  [sp_vel] -> Demux8/1
  [sp_euler] -> Demux7/1
  Demux7/2 -> [sp_pitch]
  Demux6/2 -> [sp_y]
  Demux6/3 -> [sp_z]
  [sp_rate] -> Demux9/1
  [sp_x] -> Sum/1
  [simscape_x] -> Sum/2
  Sum/1 -> PID Controller/1
  PID Controller/1 -> [cmd_effort_x]
  [simscape_y] -> Sum1/2
  Sum1/1 -> PID Controller1/1
  [sp_y] -> Sum1/1
  PID Controller1/1 -> [cmd_effort_y]
  [simscape_z] -> Sum2/2
  Sum2/1 -> PID Controller2/1
  [sp_z] -> Sum2/1
  PID Controller3/1 -> [cmd_effort_roll]
  [simscape_roll] -> Sum3/2
  PID Controller5/1 -> [cmd_effort_yaw]
  [sp_yaw] -> Sum5/1
  [simscape_yaw] -> Sum5/2
  PID Controller4/1 -> [cmd_effort_pitch]
  [sp_pitch] -> Sum4/1
  Sum4/1 -> PID Controller4/1
  Sum3/1 -> PID Controller3/1
  Sum5/1 -> PID Controller5/1
  [simscape_pitch] -> Sum4/2
  [sp_roll] -> Sum3/1
  K_pos_alpha/1 -> [K_pos_alpha]
  K_att_alpha/1 -> [K_att_alpha]
  Memory2/1 -> Demux2/1
  Memory3/1 -> Demux3/1
  Zero-Order Hold/1 -> Memory3/1
  Zero-Order Hold1/1 -> Memory2/1
  Demux2/3 -> Gain/1
  Gain/1 -> [simscape_z]
  Integrator/1 -> Scope6/1, Goto49/1
  Demux3/1 -> [simscape_yaw]
  Demux3/2 -> [simscape_pitch]
  Demux3/3 -> [simscape_roll]
  From71/1 -> MATLAB Function2/1(out_x)
  From72/1 -> MATLAB Function2/2(out_y)
  From73/1 -> MATLAB Function2/3(yaw_curr)
  MATLAB Function2/2(pitch_sp) -> Goto53/1
  MATLAB Function2/1(roll_sp) -> Goto52/1
  Integrator1/1 -> Scope7/1, Goto50/1
  Subtract/1 -> Integrator/1
  From63/1 -> Subtract/1
  From64/1 -> Subtract1/1
  Subtract1/1 -> Integrator1/1
  From74/1 -> Product6/1
  Product6/1 -> Subtract/2
  From75/1 -> Product7/1
  Product7/1 -> Subtract1/2
  Constant4/1 -> Product6/2
  Constant5/1 -> Product7/2
  Sum6/1 -> PID Controller6/1
  [cmd_effort_x] -> Scope1/1, Sum6/1
  [simscape_u] -> Memory7/1
  [simscape_v] -> Memory8/1
  PID Controller7/1 -> [ay_world_cmd]
  [cmd_effort_y] -> Sum7/1
  Sum7/1 -> PID Controller7/1
  Memory7/1 -> Scope2/1, Sum6/2
  Memory8/1 -> Sum7/2
  [thrust] -> Mux/2
  [y] -> Position/2
  [x] -> Position/1
  Mux/1 -> Scope4/1
  [alpha3] -> Servo Alpha/3
  [vx] -> Velocity/1
  [vz] -> Velocity/3
  [beta3] -> Servo Beta/3
  [beta2] -> Servo Beta/2
  [z] -> Position/3
  [rate_y] -> Rate Angular/2
  [alpha4] -> Servo Alpha/4
  [yaw] -> Attitude/3
  [beta1] -> Servo Beta/1
  [cmd_thrust] -> Mux/1
  [rate_x] -> Rate Angular/1
  [beta4] -> Servo Beta/4
  [vy] -> Velocity/2
  [alpha1] -> Servo Alpha/1
  [roll] -> Attitude/1
  [pitch] -> Attitude/2
  [alpha2] -> Servo Alpha/2
  [rate_z] -> Rate Angular/3
  From53/1 -> MATLAB Function3/1(ax_world)
  From54/1 -> MATLAB Function3/2(ay_world)
  From55/1 -> MATLAB Function3/3(cmd_thrust_z)
  From56/1 -> MATLAB Function3/4(cmd_effort_roll)
  From94/1 -> MATLAB Function3/5(cmd_effort_pitch)
  From95/1 -> MATLAB Function3/6(cmd_effort_yaw)
  From96/1 -> MATLAB Function3/9(roll)
  From97/1 -> MATLAB Function3/8(pitch)
  From99/1 -> Memory9/1
  Memory9/1 -> MATLAB Function3/10(phys_alpha_hw)
  Memory10/1 -> MATLAB Function3/11(phys_beta_hw)
  From100/1 -> Memory10/1
  From98/1 -> MATLAB Function3/7(yaw)
  From101/1 -> MATLAB Function3/12(m)
  From102/1 -> MATLAB Function3/13(g)
  From103/1 -> MATLAB Function3/14(dir_alpha)
  From104/1 -> MATLAB Function3/15(dir_beta)
  From105/1 -> MATLAB Function3/16(lim_alpha), MATLAB Function3/17(lim_beta)
  MATLAB Function3/1(cmd_hw_alpha) -> Goto48/1
  MATLAB Function3/2(cmd_hw_beta) -> Goto54/1
  MATLAB Function3/3(cmd_thrust_px4) -> Goto55/1
  PID Controller6/1 -> Scope/1, [ax_world_cmd]
  MATLAB Function1/1(cmd_hw_alpha) -> [cmd_alpha]
  MATLAB Function1/2(cmd_hw_beta) -> [cmd_beta]
  MATLAB Function1/3(cmd_thrust) -> [cmd_thrust]
  [ax_world_cmd] -> MATLAB Function1/1(ax_world)
  [ay_world_cmd] -> MATLAB Function1/2(ay_world)
  [cmd_effort_z] -> MATLAB Function1/3(cmd_thrust_z)
  [cmd_effort_roll] -> MATLAB Function1/4(cmd_effort_roll)
  [cmd_effort_pitch] -> MATLAB Function1/5(cmd_effort_pitch)
  [cmd_effort_yaw] -> MATLAB Function1/6(cmd_effort_yaw)
  [simscape_yaw] -> MATLAB Function1/7(yaw)
  [simscape_pitch] -> MATLAB Function1/8(pitch)
  [simscape_roll] -> MATLAB Function1/9(roll)
  [SYS_MASS] -> MATLAB Function1/12(m)
  [SYS_GRAVITY] -> MATLAB Function1/13(g)
  [SYS_DIR_ALPHA] -> MATLAB Function1/14(dir_alpha)
  [SYS_DIR_BETA] -> MATLAB Function1/15(dir_beta)
  [SYS_LIM_TILT] -> MATLAB Function1/16(lim_alpha), MATLAB Function1/17(lim_beta)
  [SYS_COAX_EFF] -> MATLAB Function1/19(eta_c)
  [SYS_COAX_TQ_EFF] -> MATLAB Function1/20(lam_c)
  [SYS_KQ] -> MATLAB Function1/21(c_q)
  [SYS_DIR_MOTOR_TOP] -> MATLAB Function1/22(dir_top)
  [SYS_LIM_THRUST] -> MATLAB Function1/23(max_thrust)
  [SYS_R_MAT] -> MATLAB Function1/18(R_mat)
  Memory1/1 -> MATLAB Function1/10(phys_alpha_hw)
  [phys_alpha] -> Memory1/1
  [phys_beta] -> Memory4/1
  Memory4/1 -> MATLAB Function1/11(phys_beta_hw)
  PID Controller2/1 -> Scope5/1, [cmd_effort_z]

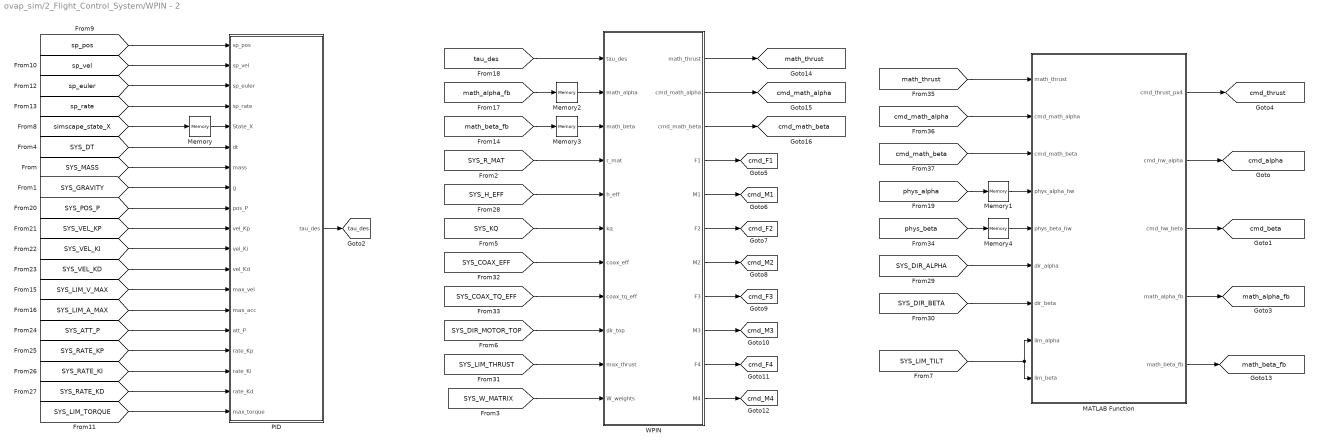
== system ovap_sim/2_Flight_Control_System/WPIN - 2 ==
  MATLAB Function : MATLAB Function  TreatAsAtomicUnit=on
  Memory{,1..4} (5 alike) : Memory
  PID : MATLAB Function  TreatAsAtomicUnit=on
  WPIN : MATLAB Function  TreatAsAtomicUnit=on
  tag scope: cmd_F1=global, cmd_F2=global, cmd_F3=global, cmd_F4=global, cmd_M1=global, cmd_M2=global, cmd_M3=global, cmd_M4=global, cmd_alpha=global, cmd_beta=global, cmd_math_alpha=global, cmd_math_beta=global, cmd_thrust=global, math_alpha_fb=global, math_beta_fb=global, math_thrust=global, tau_des=global
  wires:
  Memory/1 -> PID/5(State_X)
  [SYS_DIR_MOTOR_TOP] -> WPIN/9(dir_top)
  [SYS_RATE_KI] -> PID/17(rate_Ki)
  [SYS_VEL_KP] -> PID/10(vel_Kp)
  [SYS_MASS] -> PID/7(mass)
  [math_beta_fb] -> Memory3/1
  [SYS_LIM_TORQUE] -> PID/19(max_torque)
  [SYS_VEL_KI] -> PID/11(vel_Ki)
  [cmd_math_alpha] -> MATLAB Function/2(cmd_math_alpha)
  MATLAB Function/5(math_beta_fb) -> [math_beta_fb]
  [SYS_GRAVITY] -> PID/8(g)
  Memory4/1 -> MATLAB Function/5(phys_beta_hw)
  [SYS_KQ] -> WPIN/6(kq)
  [phys_alpha] -> Memory1/1
  WPIN/3(cmd_math_beta) -> [cmd_math_beta]
  [SYS_DIR_ALPHA] -> MATLAB Function/6(dir_alpha)
  MATLAB Function/3(cmd_hw_beta) -> [cmd_beta]
  WPIN/1(math_thrust) -> [math_thrust]
  MATLAB Function/2(cmd_hw_alpha) -> [cmd_alpha]
  [SYS_COAX_EFF] -> WPIN/7(coax_eff)
  WPIN/5(M1) -> [cmd_M1]
  [SYS_COAX_TQ_EFF] -> WPIN/8(coax_tq_eff)
  [SYS_H_EFF] -> WPIN/5(h_eff)
  [math_thrust] -> MATLAB Function/1(math_thrust)
  [tau_des] -> WPIN/1(tau_des)
  WPIN/9(M3) -> [cmd_M3]
  [SYS_LIM_THRUST] -> WPIN/10(max_thrust)
  [simscape_state_X] -> Memory/1
  [sp_pos] -> PID/1(sp_pos)
  [SYS_LIM_TILT] -> MATLAB Function/8(lim_alpha), MATLAB Function/9(lim_beta)
  [sp_euler] -> PID/3(sp_euler)
  [cmd_math_beta] -> MATLAB Function/3(cmd_math_beta)
  [SYS_LIM_A_MAX] -> PID/14(max_acc)
  WPIN/11(M4) -> [cmd_M4]
  Memory2/1 -> WPIN/2(math_alpha)
  [SYS_W_MATRIX] -> WPIN/11(W_weights)
  Memory3/1 -> WPIN/3(math_beta)
  WPIN/8(F3) -> [cmd_F3]
  WPIN/10(F4) -> [cmd_F4]
  [sp_vel] -> PID/2(sp_vel)
  WPIN/6(F2) -> [cmd_F2]
  [SYS_RATE_KD] -> PID/18(rate_Kd)
  [SYS_RATE_KP] -> PID/16(rate_Kp)
  [SYS_DT] -> PID/6(dt)
  PID/1(tau_des) -> [tau_des]
  [SYS_VEL_KD] -> PID/12(vel_Kd)
  MATLAB Function/4(math_alpha_fb) -> [math_alpha_fb]
  [phys_beta] -> Memory4/1
  [SYS_POS_P] -> PID/9(pos_P)
  [SYS_DIR_BETA] -> MATLAB Function/7(dir_beta)
  WPIN/7(M2) -> [cmd_M2]
  WPIN/4(F1) -> [cmd_F1]
  [sp_rate] -> PID/4(sp_rate)
  Memory1/1 -> MATLAB Function/4(phys_alpha_hw)
  [SYS_ATT_P] -> PID/15(att_P)
  WPIN/2(cmd_math_alpha) -> [cmd_math_alpha]
  [math_alpha_fb] -> Memory2/1
  [SYS_LIM_V_MAX] -> PID/13(max_vel)
  MATLAB Function/1(cmd_thrust_px4) -> [cmd_thrust]
  [SYS_R_MAT] -> WPIN/4(r_mat)

== matlab function ovap_sim/1_Mission_Planner/MATLAB Function ==
  settings: updateMethod=DISCRETE
  data: t input; v_max input; a_max input; w_max input; alpha_max input; dt input; sp_pos output; sp_vel output; sp_euler output; sp_rate output
function [sp_pos, sp_vel, sp_euler, sp_rate] = Mission_Planner(t, v_max, a_max, w_max, alpha_max, dt)
    % [MỚI] Thêm đầu vào 'planner_mode' để chọn chế độ hoạt động:
    % 0: Mode Tune PID (Hàm nấc - Step Response)
    % 1: Mode Bay thực tế (Kinematic Trajectory Generator)
    
    persistent traj_pos traj_vel traj_euler traj_rate
    if isempty(traj_pos)
        traj_pos = zeros(3,1); traj_vel = zeros(3,1);
        traj_euler = zeros(3,1); traj_rate = zeros(3,1);
    end

    % =====================================================================
    % 1. MISSION MANAGER (Tạo tọa độ mục tiêu thô)
    % =====================================================================
    target_pos   = [0; 0; 0];
    target_euler = [0; 0; 0];
    planner_mode = 1;

    if t < 5.0
        target_pos = [0; 0; 5.0]; 
    elseif t < 10.0
        target_pos = [10; 0; 5.0]; 
    elseif t < 20.0
        target_pos = [0; 0; 10.0]; 
    elseif t < 30.0
        target_pos = [0; 0; 10.0]; 
    else
        target_pos = [100; 0; 10.0]; 
    end
    
    % Chuyển đổi sang Radian và Cuộn setpoint Yaw về chuẩn [-pi, pi]
    target_euler = target_euler * (pi / 180);
    target_euler(3) = mod(target_euler(3) + pi, 2*pi) - pi;

    % =====================================================================
    % 2. TRAJECTORY PLANNER (Bộ tạo quỹ đạo 2 Chế độ)
    % =====================================================================
    if planner_mode == 0
        % -----------------------------------------------------------------
        % [MODE 0]: HÀM NẤC (STEP RESPONSE) - DÙNG ĐỂ TUNE PID
        % -----------------------------------------------------------------
        traj_pos   = target_pos;
        traj_euler = target_euler;
        traj_vel   = zeros(3,1);
        traj_rate  = zeros(3,1);
        
    else
        % -----------------------------------------------------------------
        % [MODE 1]: LÀM MƯỢT ĐỘNG HỌC (KINEMATIC SMOOTHING)
        % -----------------------------------------------------------------
        % Hệ số P của quỹ đạo: Độ gắt khi kéo về đích. 
        % (Không nên để quá to, máy bay sẽ thắng gấp gây lố quỹ đạo)
        k_pos_smooth = 1.0; 
        k_att_smooth = 1.0; 
        
        % --- Làm mượt Vị trí (Giới hạn Vận tốc & Gia tốc) ---
        for i = 1:3
            % B1: Tính Vận tốc mong muốn (Dùng hàm tanh tạo đường cong S)
            pos_err = target_pos(i) - traj_pos(i);
            v_target = v_max(i) * tanh((k_pos_smooth * pos_err) / v_max(i));
            
            % B2: Tính Gia tốc cần thiết để đạt v_target
            a_req = (v_target - traj_vel(i)) / dt;
            
            % B3: Bão hòa (Clamp) Gia tốc theo giới hạn phần cứng a_max
            a_req = max(min(a_req, a_max(i)), -a_max(i));
            
            % B4: Tích phân động học (Euler Integration)
            traj_vel(i) = traj_vel(i) + a_req * dt;
            traj_pos(i) = traj_pos(i) + traj_vel(i) * dt;
        end
        
        % --- Làm mượt Tư thế (Giới hạn Vận tốc góc & Gia tốc góc) ---
        for k = 1:3
            % Xử lý Shortest Path chuẩn PX4 cho Yaw
            if k == 3
                ang_err = target_euler(3) - traj_euler(3);
                ang_err = mod(ang_err + pi, 2*pi) - pi;
            else
                ang_err = target_euler(k) - traj_euler(k);
            end
            
            % B1: Tính Tốc độ góc mong muốn
            rate_target = w_max(k) * tanh((k_att_smooth * ang_err) / w_max(k));
            
            % B2: Tính Gia tốc góc cần thiết
            alpha_req = (rate_target - traj_rate(k)) / dt;
            
            % B3: Bão hòa (Clamp) Gia tốc góc theo giới hạn alpha_max
            alpha_req = max(min(alpha_req, alpha_max(k)), -alpha_max(k));
            
            % B4: Tích phân động học
            traj_rate(k)  = traj_rate(k) + alpha_req * dt;
            traj_euler(k) = traj_euler(k) + traj_rate(k) * dt;
            
            % Bọc lại góc Yaw sau khi tích phân để tránh tràn số
            if k == 3
                traj_euler(3) = mod(traj_euler(3) + pi, 2*pi) - pi;
            end
        end
    end
    
    % =====================================================================
    % 3. XUẤT TÍN HIỆU
    % =====================================================================
    sp_pos   = traj_pos; 
    sp_vel   = traj_vel;
    sp_euler = traj_euler; 
    sp_rate  = traj_rate;
end
